simulink library "libbha_kinetic_cc"  (R2013b)
settings: Solver=FixedStepDiscrete  StartTime=0.0  StopTime=Inf  FixedStep=0.004  RelTol=1e-3
PostLoadFcn:
  | , if any(exist('dsrtsu_mdlpostloadfcn', 'file') == [2, 3, 6]), try dsrtsu_mdlpostloadfcn('Execute', bdroot); catch fprintf('Error in PostLoadFcn (dsrtsu_mdlpostloadfcn) for model "%s":\n %s\n', bdroot, lasterr); end, end,
libraries: libbha_parts_bellows x2
(part 1 of 4)
settings Model: DSRTSU_INTERNAL_RTI_VER=440  DSRTSU_INTERNAL_RTI_TYPE=rti1007  DSRTSU_INTERNAL_RTIFPGA=30  Creator=Falkenhahn  LastModifiedBy=isysfalkenhahn

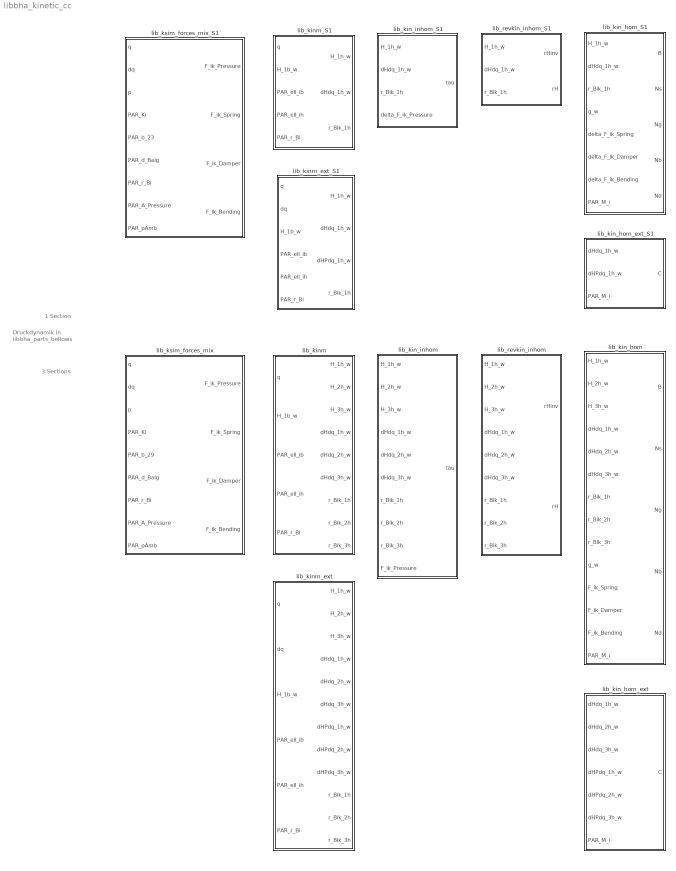
== system libbha_kinetic_cc ==
  note: Druckdynamik in
      | libbha_parts_bellows
  note: 3 Sections
  note: 1 Section
  lib_kin_hom : MATLAB Function  TreatAsAtomicUnit=on
  lib_kin_hom_S1 : MATLAB Function  TreatAsAtomicUnit=on
  lib_kin_hom_ext : MATLAB Function  TreatAsAtomicUnit=on
  lib_kin_hom_ext_S1 : MATLAB Function  TreatAsAtomicUnit=on
  lib_kin_inhom : MATLAB Function  TreatAsAtomicUnit=on
  lib_kin_inhom_S1 : MATLAB Function  TreatAsAtomicUnit=on
  lib_kinm : MATLAB Function  TreatAsAtomicUnit=on
  lib_kinm_S1 : MATLAB Function  TreatAsAtomicUnit=on
  lib_kinm_ext : MATLAB Function  TreatAsAtomicUnit=on
  lib_kinm_ext_S1 : MATLAB Function  TreatAsAtomicUnit=on
  lib_ksim_forces_mix : Subsystem
  lib_ksim_forces_mix_S1 : Subsystem
  lib_revkin_inhom : MATLAB Function  TreatAsAtomicUnit=on
  lib_revkin_inhom_S1 : MATLAB Function  TreatAsAtomicUnit=on

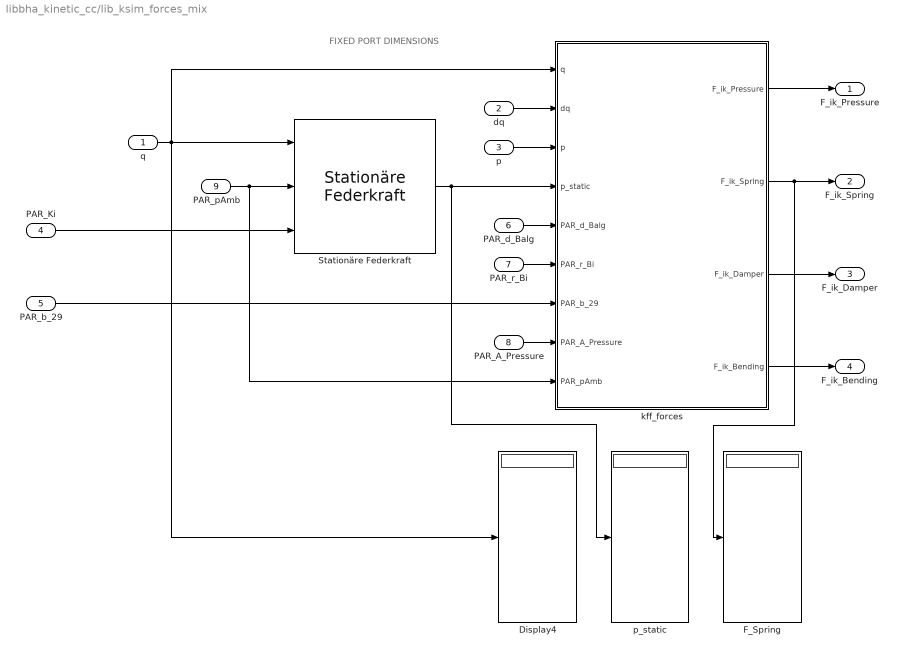
== system libbha_kinetic_cc/lib_ksim_forces_mix ==
  note: FIXED PORT DIMENSIONS
  q : Inport  PortDimensions=9
  dq : Inport  Port=2  PortDimensions=9
  p : Inport  Port=3  PortDimensions=9
  PAR_Ki : Inport  Port=4
      settings: AttributesFormatString=|
      | Parametermatrix mit Koeffizienten
      | für Federkraftinterpolation
      | 
      | 4 Spalten mit p0 p1 p2 p3
      | n Zeilen (für jeden Balg)
  PAR_b_29 : Inport  Port=5
      settings: AttributesFormatString=|
      | Parametermatrix mit linearen
      | Koeffizienten für Biegekraftinterpolation
      | 
      | 9 Spalten für 3 Sektionen/3 Bälge
      | 2 Zeilen (Einzelbalg, Doppelbalg)
  PAR_d_Balg : Inport  Port=6
  PAR_r_Bi : Inport  Port=7
  PAR_A_Pressure : Inport  Port=8
  PAR_pAmb : Inport  Port=9  PortDimensions=1
  Display4 : Display
  F_Spring : Display
  Stationäre Federkraft : libbha_parts_bellows/Stationäre Federkraft
  kff_forces : MATLAB Function  TreatAsAtomicUnit=on
  p_static : Display
  F_ik_Pressure : Outport  PortDimensions=9
  F_ik_Spring : Outport  Port=2  PortDimensions=9
  F_ik_Damper : Outport  Port=3  PortDimensions=9
  F_ik_Bending : Outport  Port=4  PortDimensions=9
  wires:
  PAR_b_29/1 -> kff_forces/7(PAR_b_29)
  PAR_r_Bi/1 -> kff_forces/6(PAR_r_Bi)
  kff_forces/4(F_ik_Bending) -> F_ik_Bending/1
  PAR_pAmb/1 -> kff_forces/9(PAR_pAmb), Stationäre Federkraft/2
  q/1 -> Display4/1, kff_forces/1(q), Stationäre Federkraft/1
  PAR_A_Pressure/1 -> kff_forces/8(PAR_A_Pressure)
  PAR_d_Balg/1 -> kff_forces/5(PAR_d_Balg)
  p/1 -> kff_forces/3(p)
  dq/1 -> kff_forces/2(dq)
  Stationäre Federkraft/1 -> kff_forces/4(p_static), p_static/1
  kff_forces/3(F_ik_Damper) -> F_ik_Damper/1
  kff_forces/2(F_ik_Spring) -> F_ik_Spring/1, F_Spring/1
  kff_forces/1(F_ik_Pressure) -> F_ik_Pressure/1
  PAR_Ki/1 -> Stationäre Federkraft/3

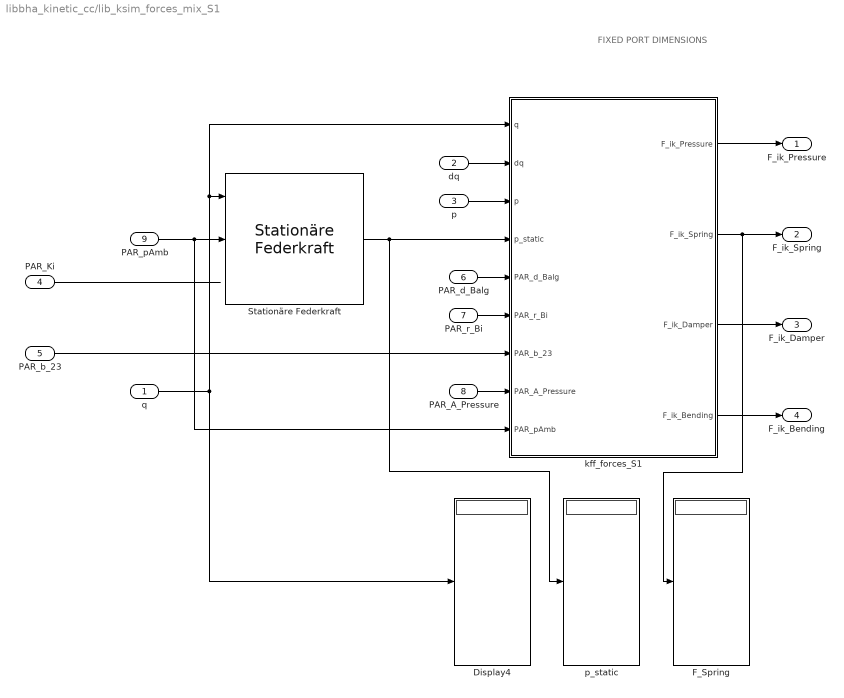
== system libbha_kinetic_cc/lib_ksim_forces_mix_S1 ==
  note: FIXED PORT DIMENSIONS
  q : Inport  PortDimensions=3
  dq : Inport  Port=2  PortDimensions=3
  p : Inport  Port=3  PortDimensions=3
  PAR_Ki : Inport  Port=4
      settings: AttributesFormatString=|
      | Parametermatrix mit Koeffizienten
      | für Federkraftinterpolation
      | 
      | 4 Spalten mit p0 p1 p2 p3
      | n Zeilen (für jeden Balg)
  PAR_b_23 : Inport  Port=5  PortDimensions=1
      settings: AttributesFormatString=|
      | Parametermatrix mit linearen
      | Koeffizienten für Biegekraftinterpolation
      | 
      | 9 Spalten für 3 Sektionen/3 Bälge
      | 2 Zeilen (Einzelbalg, Doppelbalg)
  PAR_d_Balg : Inport  Port=6  PortDimensions=1
  PAR_r_Bi : Inport  Port=7  PortDimensions=1
  PAR_A_Pressure : Inport  Port=8  PortDimensions=1
  PAR_pAmb : Inport  Port=9  PortDimensions=1
  Display4 : Display
  F_Spring : Display
  Stationäre Federkraft : libbha_parts_bellows/Stationäre Federkraft
  kff_forces_S1 : MATLAB Function  TreatAsAtomicUnit=on
  p_static : Display
  F_ik_Pressure : Outport  PortDimensions=3
  F_ik_Spring : Outport  Port=2  PortDimensions=3
  F_ik_Damper : Outport  Port=3  PortDimensions=3
  F_ik_Bending : Outport  Port=4  PortDimensions=3
  wires:
  kff_forces_S1/1(F_ik_Pressure) -> F_ik_Pressure/1
  kff_forces_S1/2(F_ik_Spring) -> F_Spring/1, F_ik_Spring/1
  kff_forces_S1/3(F_ik_Damper) -> F_ik_Damper/1
  Stationäre Federkraft/1 -> p_static/1, kff_forces_S1/4(p_static)
  dq/1 -> kff_forces_S1/2(dq)
  p/1 -> kff_forces_S1/3(p)
  PAR_d_Balg/1 -> kff_forces_S1/5(PAR_d_Balg)
  PAR_A_Pressure/1 -> kff_forces_S1/8(PAR_A_Pressure)
  q/1 -> kff_forces_S1/1(q), Stationäre Federkraft/1, Display4/1
  PAR_pAmb/1 -> kff_forces_S1/9(PAR_pAmb), Stationäre Federkraft/2
  kff_forces_S1/4(F_ik_Bending) -> F_ik_Bending/1
  PAR_r_Bi/1 -> kff_forces_S1/6(PAR_r_Bi)
  PAR_b_23/1 -> kff_forces_S1/7(PAR_b_23)
  PAR_Ki/1 -> ?

== matlab function libbha_kinetic_cc/lib_kinm_S1 ==
  data: q input size=[3,1]; H_1b_w input size=[4,4]; PAR_ell_ib input size=1; PAR_ell_ih input size=1; PAR_r_Bi input size=1; H_1h_w output size=[4,4]; dHdq_1h_w output size=[12,4]; r_Bik_1h output size=[4,3]
function [H_1h_w, dHdq_1h_w, r_Bik_1h] =  ksim_kinematic( q, H_1b_w,PAR_ell_ib,PAR_ell_ih, PAR_r_Bi)


%% Zustands- und Ableitungsberechnung der Homogenen Transformationen
    
    k                 = calc_k_i(q(1), q(2), q(3), PAR_r_Bi(1));
    
    dkdq_S1              = calc_dkdq_i(q(1), q(2), q(3), PAR_r_Bi(1));
    
    % Relative Homogene Transformation und dessen Ableitung im lokalen Sektions-KoSy    
	[H_1h_1b, H_1b1, H_1h1] = calc_H_ih_ib(k(1), k(2), k(3), PAR_ell_ib(1), PAR_ell_ih(1));
    
    [dHdq_1h_1b, ~] = calc_dHdq_ih_ib(k(1), k(2), k(3), dkdq_S1, H_1b1, H_1h1);
    
    % Absolute Homogene Transformation und dessen Ableitung im Welt-KoSy
    H_1h_w = H_1b_w * H_1h_1b;
    
    dHdq_1h_w = zeros(4*3,4); % 4x4 Matrix abgeleitet nach 3 Zuständen q_i. 
    dHdq_1h_w((1:12)   ,:) = MM(H_1b_w,dHdq_1h_1b);
	
%% Kinetische Vorwärtsrechnung

    %r_S1_1h = [0;0;0;1];
    %r_S2_2h = [0;0;0;1];
    %r_S3_3h = [0;0;0;1];
    
    r_Bik_1h = [ PAR_r_Bi(1), -PAR_r_Bi(1)/2,         -PAR_r_Bi(1)/2;
				 0,            sqrt(3)/2*PAR_r_Bi(1),  -sqrt(3)/2*PAR_r_Bi(1)  
                 0, 0, 0; 1, 1, 1 ];

end

% ##################### Hilfsfunktionen #####################

%%  Konfigurationszustand k = [phi, kappa, ell]^T 

%  Konfigurationszustand einer Sektion 
function [k_i] = calc_k_i(q1,q2,q3, d)
    % Input:
    %   - qi = [ell_i1, ell_i2, ell_i3]^T       Aktorzustand
    %   - d                                     Radialer Abstand der Aktorsymmetrielinie  
    %
    % Output:
    %   - ki   [3 x 1]                          Konfigurationszustand 

    % Vermeidung Singularität
    qist_eps  = 1e-15;
    qist      = q1.^2 + q2.^2 + q3.^2 - q1.*q2 - q1.*q3 - q2.*q3;
    while (qist<qist_eps)
        q1      = q1 - 5e-8;
        qist  = q1.^2 + q2.^2 + q3.^2 - q1.*q2 - q1.*q3 - q2.*q3;
    end

    % Substitutionen
    q_sum   = q1 + q2 + q3;
    
    % Konfigurationszustand
    mphi    = atan2(sqrt(0.3e1) * (q3-q2) , (q2+q3 - 2*q1));
    mkappa  = 2.0 * sqrt(qist) / (d*q_sum);
    mell    = (q1 + q2 + q3)/3.0;
    
    k_i = [mphi;
           mkappa;
           mell];
end

% Partielle Ableitung 1. Ordnung nach q
function [dkdq_i] = calc_dkdq_i(q1,q2,q3, d)

    % Input:
	%   - qi = [ell_i1, ell_i2, ell_i3]^T       Aktorzustand
    %   - d                                     Radialer Abstand der Aktorsymmetrielinie
	%
	% Output:
	%   - dkdq_i   [3 x 3]                      Partielle Ableitung von Konfigurationszuständen ki nach Aktorzuständen qi 
 
    % Vermeidung Singularität
    qist_eps  = 1e-15;
    qist      = q1.^2 + q2.^2 + q3.^2 - q1.*q2 - q1.*q3 - q2.*q3;
    while (qist<qist_eps)
        q1      = q1-5e-8;
        qist  = q1.^2 + q2.^2 + q3.^2 - q1*q2 - q1*q3 - q2*q3;
    end

    % Substitutionen
    q_sum   = q1 + q2 + q3;

    % Ableitungen
    dkdq_i = zeros(3, 3);
    
    % dk1_dqb
    mdphi_dq1 =  sqrt(3.0) * ( q3 - q2) / qist / 2.0;
    mdphi_dq2 =  sqrt(3.0) * (-q3 + q1) / qist / 2.0;
    mdphi_dq3 = -sqrt(3.0) * (-q2 + q1) / qist / 2.0;
    
    dkdq_i(1, :) = [mdphi_dq1, mdphi_dq2, mdphi_dq3];
    
    % dk2_dqb
    mdkappa_dq1 =  3 * ( q2*q1 - q2^2  + q3*q1 - q3^2) / sqrt(qist) / d / q_sum^2;
    mdkappa_dq2 = -3 * (-q2*q1 - q2*q3 + q3^2  + q1^2) / sqrt(qist) / d / q_sum^2;
    mdkappa_dq3 = -3 * ( q2^2  - q2*q3 - q3*q1 + q1^2) / sqrt(qist) / d / q_sum^2;
    
    dkdq_i(2, :) = [mdkappa_dq1, mdkappa_dq2, mdkappa_dq3];
    
    % dk3_dqb
    mdell_dq1 = 1.0/3.0;
    mdell_dq2 = 1.0/3.0;
    mdell_dq3 = 1.0/3.0;
    
    dkdq_i(3, :) = [mdell_dq1, mdell_dq2, mdell_dq3];
end

%%  Homogene Transformationen 

%  Homogene Transformation 
%function [H_ih_ib] = calc_H_ih_ib(k1, k2, k3, PAR_ell_ib, PAR_ell_ih) 
function [H_ih_ib, H_im1_ib, H_ih_i] = calc_H_ih_ib(k1, k2, k3, PAR_ell_ib, PAR_ell_ih) 
    % Input:
    %   - ki = [phi, kappa, ell]^T              Konfigurationszustand
    %
    % Output:
    %   - H_i_im1   [4 x 4]                     Homogene Transformation
    
    % Vermeidung Singularität
    k2_eps = 1e-6;
    k2     = max([k2_eps, k2]);
    
    % Substitutionen
    sk1     = sin(k1);
    ck1     = cos(k1);
    sk2k3   = sin(k2 * k3);
    ck2k3   = cos(k2 * k3);
    
    % Trafo
    mHT_i_im1_11 = ck1 ^ 2 * (ck2k3 - 0.1e1) + 0.1e1;
    mHT_i_im1_12 = sk1 * ck1 * (ck2k3 - 0.1e1);
    mHT_i_im1_13 = ck1 * sk2k3;
    mHT_i_im1_14 = -ck1 * (ck2k3 - 0.1e1) / k2;
    
    mHT_i_im1_21 = sk1 * ck1 * (ck2k3 - 0.1e1);
    mHT_i_im1_22 = -ck1 ^ 2 * (ck2k3 - 0.1e1) + ck2k3;
    mHT_i_im1_23 = sk1 * sk2k3;
    mHT_i_im1_24 = -sk1 * (ck2k3 - 0.1e1) / k2;
    
    mHT_i_im1_31 = -ck1 * sk2k3;
    mHT_i_im1_32 = -sk1 * sk2k3;
    mHT_i_im1_33 = ck2k3;
    mHT_i_im1_34 = sk2k3 / k2;
    
    H_i_im1 = [mHT_i_im1_11, mHT_i_im1_12, mHT_i_im1_13, mHT_i_im1_14;
               mHT_i_im1_21, mHT_i_im1_22, mHT_i_im1_23, mHT_i_im1_24;
               mHT_i_im1_31, mHT_i_im1_32, mHT_i_im1_33, mHT_i_im1_34;
               0,            0,            0,            1            ];
           
    % Statische Begrenzungen
    H_im1_ib = eye(4);    
    H_ih_i   = eye(4);
    H_im1_ib(3,4) = PAR_ell_ib;
	H_ih_i(3,4)   = PAR_ell_ih;
    
    H_ih_ib = H_im1_ib * H_i_im1 * H_ih_i;
end

function [dHdk_i_i] = calc_dHdk_i_i(k1, k2, k3)
    % Input:
	%   - ki = [phi, kappa, ell]^T              Konfigurationszustand
	%
	% Output:
	%   - dH_i_in_im1_dka   [4*3x4]      Partielle Ableitung von H_i_in_im1 nach allen Konfigurationszuständen ki mit dim_ki=3
    
    % Vermeidung Singularität
    k2_eps = 1e-6;
    k2     = max([k2_eps, k2]);
    
    % Substitutionen
    sk1     = sin(k1);
    ck1     = cos(k1);
    sk2k3   = sin(k2 * k3);
    ck2k3   = cos(k2 * k3);
    
    dHdk_i_i = zeros(4*3, 4);
    
    % dHdk1_i_im1
    mdH_i_in_im1_dk1_11 = -2 * sk1 * ck1 * (ck2k3 - 1);
    mdH_i_in_im1_dk1_12 = 2 * ck2k3 * ck1 ^ 2 - ck2k3 - 2 * ck1 ^ 2 + 1;
    mdH_i_in_im1_dk1_13 = -sk1 * sk2k3;
    mdH_i_in_im1_dk1_14 = sk1 * (ck2k3 - 1) / k2;
    
    mdH_i_in_im1_dk1_21 = 2 * ck2k3 * ck1 ^ 2 - ck2k3 - 2 * ck1 ^ 2 + 1;
    mdH_i_in_im1_dk1_22 = 2 * sk1 * ck1 * (ck2k3 - 1);
    mdH_i_in_im1_dk1_23 = ck1 * sk2k3;
    mdH_i_in_im1_dk1_24 = -ck1 * (ck2k3 - 1) / k2;
    
    mdH_i_in_im1_dk1_31 = sk1 * sk2k3;
    mdH_i_in_im1_dk1_32 = -ck1 * sk2k3;
    mdH_i_in_im1_dk1_33 = 0;
    mdH_i_in_im1_dk1_34 = 0;
    
    dHdk_i_i(1:3,:) =         [mdH_i_in_im1_dk1_11, mdH_i_in_im1_dk1_12, mdH_i_in_im1_dk1_13, mdH_i_in_im1_dk1_14;
                               mdH_i_in_im1_dk1_21, mdH_i_in_im1_dk1_22, mdH_i_in_im1_dk1_23, mdH_i_in_im1_dk1_24;
                               mdH_i_in_im1_dk1_31, mdH_i_in_im1_dk1_32, mdH_i_in_im1_dk1_33, mdH_i_in_im1_dk1_34 ];
    
    % dHdk2_i_im1
    mdH_i_in_im1_dk2_11 = -ck1 ^ 2 * sk2k3 * k3;
    mdH_i_in_im1_dk2_12 = -sk1 * ck1 * sk2k3 * k3;
    mdH_i_in_im1_dk2_13 = ck1 * ck2k3 * k3;
    mdH_i_in_im1_dk2_14 = ck1 * (sk2k3 * k3 * k2 + ck2k3 - 1) / k2 ^ 2;
    
    mdH_i_in_im1_dk2_21 = -sk1 * ck1 * sk2k3 * k3;
    mdH_i_in_im1_dk2_22 = -sk2k3 * sk1 ^ 2 * k3;
    mdH_i_in_im1_dk2_23 = sk1 * ck2k3 * k3;
    mdH_i_in_im1_dk2_24 = sk1 * (sk2k3 * k3 * k2 + ck2k3 - 1) / k2 ^ 2;
    
    mdH_i_in_im1_dk2_31 = -ck1 * ck2k3 * k3;
    mdH_i_in_im1_dk2_32 = -sk1 * ck2k3 * k3;
    mdH_i_in_im1_dk2_33 = -sk2k3 * k3;
    mdH_i_in_im1_dk2_34 = (ck2k3 * k3 * k2 - sk2k3) / k2 ^ 2;
    
    dHdk_i_i(5:7,:) =         [mdH_i_in_im1_dk2_11, mdH_i_in_im1_dk2_12, mdH_i_in_im1_dk2_13, mdH_i_in_im1_dk2_14;
                               mdH_i_in_im1_dk2_21, mdH_i_in_im1_dk2_22, mdH_i_in_im1_dk2_23, mdH_i_in_im1_dk2_24;
                               mdH_i_in_im1_dk2_31, mdH_i_in_im1_dk2_32, mdH_i_in_im1_dk2_33, mdH_i_in_im1_dk2_34 ];
    
    % dHdk3_i_im1
    mdH_i_in_im1_dk3_11 = -ck1 ^ 2 * sk2k3 * k2;
    mdH_i_in_im1_dk3_12 = -sk1 * ck1 * sk2k3 * k2;
    mdH_i_in_im1_dk3_13 = ck1 * ck2k3 * k2;
    mdH_i_in_im1_dk3_14 = ck1 * sk2k3;
    
    mdH_i_in_im1_dk3_21 = -sk1 * ck1 * sk2k3 * k2;
    mdH_i_in_im1_dk3_22 = -sk2k3 * sk1 ^ 2 * k2;
    mdH_i_in_im1_dk3_23 = sk1 * ck2k3 * k2;
    mdH_i_in_im1_dk3_24 = sk1 * sk2k3;
    
    mdH_i_in_im1_dk3_31 = -ck1 * ck2k3 * k2;
    mdH_i_in_im1_dk3_32 = -sk1 * ck2k3 * k2;
    mdH_i_in_im1_dk3_33 = -sk2k3 * k2;
    mdH_i_in_im1_dk3_34 = ck2k3;
    
    dHdk_i_i(9:11,:) =        [mdH_i_in_im1_dk3_11, mdH_i_in_im1_dk3_12, mdH_i_in_im1_dk3_13, mdH_i_in_im1_dk3_14;
                               mdH_i_in_im1_dk3_21, mdH_i_in_im1_dk3_22, mdH_i_in_im1_dk3_23, mdH_i_in_im1_dk3_24;
                               mdH_i_in_im1_dk3_31, mdH_i_in_im1_dk3_32, mdH_i_in_im1_dk3_33, mdH_i_in_im1_dk3_34 ];
end

%function [dHdq_ih_ib, dHdk_ih_ib] = calc_dHdq_ih_ib(k1, k2, k3, dkdq_i, PAR_ell_ib, PAR_ell_ih)
function [dHdq_ih_ib, dHdk_ih_ib] = calc_dHdq_ih_ib(k1, k2, k3, dkdq_i, H_ibi, H_ihi)

    % Input:
	%   - ki = [phi, kappa, ell]^T              Konfigurationszustand
	%   - dkdq_i            [3=dim_kix3=dim_qi] Partielle Ableitung von allen Konfigurationszuständen ki nach allen Aktorzuständen qi 
	%
	% Output:
	%   - dH_i_in_im1_dqa   [4*3x4]      Partielle Ableitung von H_ih_ib nach allen Aktorzuständen qi mit dim_di = 3

    dHdq_ih_ib = zeros(4*3,4);

    % Statische Begrenzungen
    %H_im1_ib = eye(4);    
    %H_ih_i   = eye(4);
    %H_im1_ib(3,4) = PAR_ell_ib;
	%H_ih_i(3,4)   = PAR_ell_ih;
    
    % Kettenregel
    dHdk_ih_ib = calc_dHdk_i_i(k1, k2, k3);
    for j=1:3
		jm = j-1;
		%dHdq_ih_ib((1:4)+jm*4,:) = H_im1_ib * (dHdk_ih_ib(1:4,:).*dkdq_i(1,j) + dHdk_ih_ib(5:8,:).*dkdq_i(2,j) + dHdk_ih_ib(9:12,:).*dkdq_i(3,j)) * H_ih_i; % H_base * ( dHdq_i_i ) * H_head // mit dHdq_i_i = dH/dk1 * dk1/dqj + dH/dk2 * dk2/dqj + dH/dk3 * dk3/dqj
		dHdq_ih_ib((1:4)+jm*4,:) = H_ibi * (dHdk_ih_ib(1:4,:).*dkdq_i(1,j) + dHdk_ih_ib(5:8,:).*dkdq_i(2,j) + dHdk_ih_ib(9:12,:).*dkdq_i(3,j)) * H_ihi; % H_base * ( dHdq_i_i ) * H_head // mit dHdq_i_i = dH/dk1 * dk1/dqj + dH/dk2 * dk2/dqj + dH/dk3 * dk3/dqj
    end
end

%% Matrix Helpers

function [H_2_0] = MM(H_1_0, H_2_1) % Matrix Multiplikation für 4x4 * 4nzx4ns
	% Input:
	%   - Eine Matrix [4x4]
	%   - Eine Matrix [4*nz x 4*ns]
	%
	% Output:
	%   - H_2_in_0 [4*n x 4*ns] = H_1_in_0*H_2_in_1

	[nz1, ns1] = size(H_1_0);
	[nz2, ns2] = size(H_2_1);

	nz_max = max(nz1./4, nz2./4);
	ns_max = max(ns1./4, ns2./4);

	H_2_0 = zeros(4*nz_max, 4*ns_max);

	if (nz1+ns1) < (nz2+ns2)
		for zz = 1:nz_max
			for ss = 1:ns_max
				H_2_0((1:4)+4*(zz-1), (1:4)+4*(ss-1)) = H_1_0 * H_2_1((1:4)+4*(zz-1), (1:4)+4*(ss-1));
			end
		end
	else
		for zz = 1:nz_max
			for ss = 1:ns_max
				H_2_0((1:4)+4*(zz-1), (1:4)+4*(ss-1)) = H_1_0((1:4)+4*(zz-1), (1:4)+4*(ss-1)) * H_2_1;
			end
		end
	end
end

== matlab function libbha_kinetic_cc/lib_ksim_forces_mix/kff_forces ==
  data: q input; dq input; p input; p_static input; F_ik_Pressure output; PAR_d_Balg input size=9; PAR_r_Bi input size=3; PAR_b_29 input size=[2,9]; PAR_A_Pressure input size=9; PAR_pAmb input; F_ik_Spring output; F_ik_Damper output; F_ik_Bending output
function [F_ik_Pressure, F_ik_Spring, F_ik_Damper, F_ik_Bending]  = kff_forces(q, dq, p, p_static, PAR_d_Balg, PAR_r_Bi, PAR_b_29, PAR_A_Pressure, PAR_pAmb)
%
% Parameter
%   - [unused]          Schalter zum Definieren der Modi
%   - PAR_A_Pressure    Wirksame Fläche der Druckkraft (sektionsweise)
%   - PAR_D_Balg        Dämpfungsparameter (sektionsweise)
%   - PAR_pAmb          Umgebungsdruck

    %#codegen
    
    %% Druckkraft
    F_ik_Pressure = (p - PAR_pAmb) .* PAR_A_Pressure;
    
    %% Dämperkraft
    F_ik_Damper   = dq .* PAR_d_Balg;
    
    %% Federkraft 
    F_ik_Spring = PAR_A_Pressure.* p_static;
    
    %% Biegekraft 
    % neue Biegekraftberechnung
    k                 = [ calc_k_i(q(1), q(2), q(3), PAR_r_Bi(1)), ... % phi1   phi2   phi3
                          calc_k_i(q(4), q(5), q(6), PAR_r_Bi(2)), ... % kappa1 kappa2 kappa3
                          calc_k_i(q(7), q(8), q(9), PAR_r_Bi(3)) ];   % ell1   ell2   ell3
                      
    F_ik_Bending = fcn_getpbend(k(1,:), k(2,:), k(3,:), PAR_b_29) .* PAR_A_Pressure; 

 
end

% D:\Dokumente\Projekte\Festo-BHA\23 Messergebnisse\Federkennlinie (Identifizierung) (2015-06) ISYS
function p_bend = fcn_getpbend(phi, kappa, ell, PAR_kl_gain) 
    % phi   = [1 x n]
    % kappa = [1 x n]
    % ell   = [1 x n]
    % PAR_kl_gain = [2 x 3*n] mit [2 x 3] = [M1:1 M2:1 M3:1; M1:2 M2:2 M3:2]'
    %               (erste Zeile: Einzelbälge, zweite Zeile Doppelbälge)
    
    % vektorielle Eingänge gelten für 3 Sektionen
    % Phi muss als Spaltenvektor (eine Zeile) vorliegen
    
    %% Bestimmung der Phi-Projektion des aufgeteilten Phi-Kreises
    [iStart,iEnd,tcos] = fcn_split_phi(phi); % für jedes Phi Start- und End-Indices mit Gewichtungsverhältnis (tcos) berechnen
    % Start- und Endindex/Messzuweisung pro Sektion/Phi: 
    % abs(.) -> Messnummer (Einzelbalg i gegen restlichen Doppelbalg)
    % sign(.) -> Vorzeichen (+kappa/-kappa)
    % Kurve 1 oder 2 aus 2-(Balgnummer==abs(Messzuweisung);
    
    %% Für jede Sektion entsprechende Zeilen aus PAR_kl_gain auswählen
    %       111   121   131   211   221   231   311   321   331  <-- PAR_kl_gain
    %       112   122   132   212   222   232   312   322   332
    %       ---------------   ---------------   ---------------  <-- iStart-Index wähl von jedem Block die i-te Spalte aus
        
    valStart = PAR_kl_gain(:,abs(iStart)+(0:2)*3) .* ([1;1]*(sign(iStart).*kappa.*ell));
    valEnd   = PAR_kl_gain(:,abs(iEnd)  +(0:2)*3) .* ([1;1]*(sign(iEnd  ).*kappa.*ell)); 
    
    % Zwei Ergebnisse der beiden Parameterkurven auf drei Bälge übertragen
    % Matrix: Zeilen entsprechen den Bälgen, Spalten den Sektionen
    %   Indizierung: erster Teil Balgzuweisungen (aus 1 oder 2) pro Sektion,
    %                zweiter Teil: Skalierung auf Gesamtindices
        
    pStart   = valStart( 2-(repmat([1;2;3],1,3)-repmat(abs(iStart),3,1)==0)  +  [1;1;1]*(0:2)*2 );
    pEnd     = valEnd(   2-(repmat([1;2;3],1,3)-repmat(abs(iEnd  ),3,1)==0)  +  [1;1;1]*(0:2)*2 );
    
    delta = (pEnd - pStart)/2;
    mw    = (pEnd + pStart)/2;
    
    % Cosinus-Interpolation zwischen Start und Ende (mittels Mittelwert und Delta)
    res   = -delta.*cos([1;1;1]*tcos) + mw;
    
    p_bend = reshape(res,9,1); 
end

function [iStart,iEnd,tcos] = fcn_split_phi(phi)
    %% Rückgabe:
    %       iStart: [1xlenphi]  (früher [3xlenphi])
    %       iEnd:   [1xlenphi]  (früher [3xlenphi])
    %       tcos:   [1xlenphi] <-- ggf auch transponiert, wenn phi nicht [1xX]

    %% Aufteilung des Phi-Kreises in 6 Bereiche         Balg 1      Balg 2      Balg 3
    % 0   .. 1/3 pi  --  Krümmung zu (1)                +M1:1		+M1:2		+M1:2
    % 1/3 .. 2/3 pi  --  Krümmung zu (1-2)              -M3:2       -M3:2       -M3:1
    % 2/3 .. 1   pi  --  Krümmung zu (2)                +M2:2       +M2:1       +M2:2
    % 1   .. 4/3 pi  --  Krümmung zu (2-3)              -M1:1       -M1:2       -M1:2
    % 4/3 .. 5/3 pi  --  Krümmung zu (3)                +M3:2       +M3:2       +M3:1
    % 5/3 .. 2   pi  --  Krümmung zu (3-1)              -M2:2       -M2:1       -M2:2

    % Indexzuweisungen: jew. Messungen für verschiedene Phasen
    Messzuweisung = [ +1, -3, +2, -1, +3, -2]; % ob Kurve 1 oder 2 ergibt sich aus 2-(Balgnummer==abs(Messzuweisung);
    
    %% Cosinus-Interpolation zwischen allen Start- und Endvektoren
    % liefert Startindex (1-6) und Endindex
    tcos = mod((phi*3),pi); % arg(cos) zwischen 0 und pi
    %tcos = mod((phi/pi),1/3)*3*pi; %% gleiches Ergebnis
    
    %% Phi-abhängige Auswahl der 6 Bereiche für alle drei Bälge
    % sel_idx   = mod([1;1;1]*round((3*phi-tcos)/pi)+([1;5;3]-1)*ones(1,size(phi,2)),6)+1;   % Formel: Zeileneintrag für jeden Balg, phi muss als Zeilenvektor (horizontal) vorliegen (ein Eintrag pro Sektion)
    sel_idx   = mod(round((3*phi-tcos)/pi),6)+1;                                             % Formel: nur ein Zeileneintrag,        phi kann als Zeilenvektor (horizontal) vorliegen (ein Eintrag pro Sektion)
    
    iStart = Messzuweisung(sel_idx);
    iEnd   = Messzuweisung(mod(sel_idx,6)+1);
    
end

%%  Konfigurationszustand k = [phi, kappa, ell]^T 
% aus: libbha_kinetic_cc\lib_kinm

%  Konfigurationszustand einer Sektion 
function [k_i] = calc_k_i(q1,q2,q3, d)
    % Input:
    %   - qi = [ell_i1, ell_i2, ell_i3]^T       Aktorzustand
    %   - d                                     Radialer Abstand der Aktorsymmetrielinie  
    %
    % Output:
    %   - ki   [3 x 1]                          Konfigurationszustand 

    % Vermeidung Singularität
    qist_eps  = 1e-15;
    qist      = q1.^2 + q2.^2 + q3.^2 - q1.*q2 - q1.*q3 - q2.*q3;
    while (qist<qist_eps)
        q1      = q1 - 5e-8;
        qist  = q1.^2 + q2.^2 + q3.^2 - q1.*q2 - q1.*q3 - q2.*q3;
    end

    % Substitutionen
    q_sum   = q1 + q2 + q3;
    
    % Konfigurationszustand
    mphi    = atan2(sqrt(0.3e1) * (q3-q2) , (q2+q3 - 2*q1));
    mkappa  = 2.0 * sqrt(qist) / (d*q_sum);
    mell    = (q1 + q2 + q3)/3.0;
    
    k_i = [mphi;
           mkappa;
           mell];
end




% %% Biegekraft 
%     % Biegefeder: Biegemoment mal Biege-Bogenlänge
%     % Abgeleitet nach Bogenlänge: Biegekraft F_rot in Gelenkkoordinaten (q)
%     % (entspricht dMrot/dq)
% 
%     F_ik_Bending_q       = zeros(9,1); 
%     PAR_rot = 4/9*PAR_c_Ri./PAR_r_Bi.^2;
%     for xi = 1:3 %3 Sektionen
%         F_ik_Bending_q(3*xi-2) = PAR_rot(xi) * (2*q(3*xi-2) - q(3*xi-1) - q(3*xi-0));
%         F_ik_Bending_q(3*xi-1) = PAR_rot(xi) * (2*q(3*xi-1) - q(3*xi-2) - q(3*xi-0));
%         F_ik_Bending_q(3*xi-0) = PAR_rot(xi) * (2*q(3*xi-0) - q(3*xi-2) - q(3*xi-1));
%     end 

% ggf auslagern und in Initialisierungsfile vornehmen
% function par9 = parcon3t9(par3)
%     par9 = zeros(9,1);
%     if size(par3,1) == 3 && size(par3,2) == 1
%         par9 = reshape((par3*[1, 1, 1])',9,1);
%     elseif size(par3,1) == 1 && size(par3,2) == 3
%         par9 = reshape(([1; 1; 1;]*par3),9,1);
%     else
%         error('wrong parameter format');
%     end
% end

%% Alter Federkraftfunktionen

%  %% Federkraft aus Lookuptabelle mit linearer Extrapolation
%     % Stand 2013-11
%     % Absoluter Druck über absoluter Länge
%     
% %     % Nur quasilinearer Teil der Kennlinie ohne "auf-Block-fahren"
% %     PAR_lt_l = [0.1707;0.1755;0.1802;0.1853;0.1906;0.1961;0.2015;0.2068;0.2122;0.2175;0.2227;0.2277;0.2324;0.2371;0.2417;0.2461;0.2502;0.2544;0.2583;0.2621;0.2658;0.2695;0.2728;0.2767;0.2803];
% %     PAR_lt_p = [85064;90057;95042;100042;105031;110032;115029;120023;125016;130011;135005;140000;144995;149987;154982;159976;164974;169967;174962;179959;184959;189947;194941;199833;204790];
% %     
% %     % Steil abflachende, aufgenommene Kurve. Bei Unterdruck keine
% %     % Längenänderung mehr vorhanden
% %     PAR_lt_l = [0.16768;0.16774;0.16798;0.16811;0.16828;0.16884;0.16982;0.1707;0.1755;0.1802;0.1853;0.1906;0.1961;0.2015;0.2068;0.2122;0.2175;0.2227;0.2277;0.2324;0.2371;0.2417;0.2461;0.2502;0.2544;0.2583;0.2621;0.2658;0.2695;0.2728;0.2767;0.2803];
% %     PAR_lt_p = [55080;70074;75061;79990;81483;82985;84485;85064;90057;95042;100042;105031;110032;115029;120023;125016;130011;135005;140000;144995;149987;154982;159976;164974;169967;174962;179959;184959;189947;194941;199833;204790];
% %     
% %     p_static = zeros(9,1);
% %     for i=1:9
% %         if q(i) < PAR_lt_l(1) % Lineare Extrapolation für kleinere Werte
% %             p_static(i) = (PAR_lt_p(2) - PAR_lt_p(1))/(PAR_lt_l(2) - PAR_lt_l(1)) * (q(i) - PAR_lt_l(1)) + PAR_lt_p(1); 
% %         elseif q(i) > PAR_lt_l(end) % Lineare Extrapolation für größere Werte
% %             p_static(i) = (PAR_lt_p(end) - PAR_lt_p(end-1))/(PAR_lt_l(end) - PAR_lt_l(end-1)) * (q(i) - PAR_lt_l(end-1)) + PAR_lt_p(end-1);
% %         else
% %             p_static(i) = interp1(PAR_lt_l, PAR_lt_p, q(i), 'linear');
% %         end
% %     end
% %     F_ik_Spring = parcon3t9(PAR_A_Pressure).*(p_static - PAR_pAmb);
%     
%     %% Federkraft aus Fitfunktion (v0) [Mahl]
%     % Stand 2012-12
%     
% %     PAR_c_Balg_lin = 1e3*[4.2482;3.7425;4.0144];
% %     PAR_c_Balg_sqr = 1e4*[ 1.7658;1.6086;1.0499];
% %     delta_l = (q - parcon3t9([0.174; 0.174; 0.174]));
% %     F_ik_Spring   = delta_l .* parcon3t9(PAR_c_Balg_lin) + delta_l.^2 .* parcon3t9(PAR_c_Balg_sqr);
% 
%     %% Federkraft aus Fitfunktion (v1)
%     % Stand 2013-01
%     
% %     PAR_c_FFB5 = [ 7.453e5 -4.758e4 1.133e8 -1.797e9 9.122e9 ];
% %     delta_l = (q - parcon3t9([0.174; 0.174; 0.174]));
% %     F_ik_Spring = parcon3t9(PAR_A_Pressure).*(PAR_c_FFB5(1)*delta_l + PAR_c_FFB5(2)*delta_l.^2 + PAR_c_FFB5(3)*delta_l.^3 + PAR_c_FFB5(4)*delta_l.^4 + PAR_c_FFB5(5)*delta_l.^5);
%     
%     %% Federkraft aus Fitfunktion (v2)
%     % Stand 2013-11
%     % Absoluter Druck über absoluter Länge
%     
%     PAR_c_FFB5 = [ -1.987e+06; 3.8e+07; -2.783e+08; 1.009e+09; -1.763e+09; 1.197e+09 ];
%     PAR_pAmb = 1e5;
%     F_ik_Spring = parcon3t9(PAR_A_Pressure).*(PAR_c_FFB5(1) + PAR_c_FFB5(2)*q + PAR_c_FFB5(3)*q.^2 + PAR_c_FFB5(4)*q.^3 + PAR_c_FFB5(5)*q.^4 + PAR_c_FFB5(6)*q.^5 - PAR_pAmb);
%
